simulink model "massignment5"  (Simulink 6.0)
settings: Solver=FixedStepDiscrete  StartTime=0.0  StopTime=10.0  RelTol=1e-3
libraries: massignmentLib x2
settings Model: Creator=awarlock  LastModifiedBy=awarlock  ExtModeAutoUpdateStatusClock=off
settings OptimizationCC: InlineParams=on
settings DebuggingCC: MultiTaskDSMMsg=warning

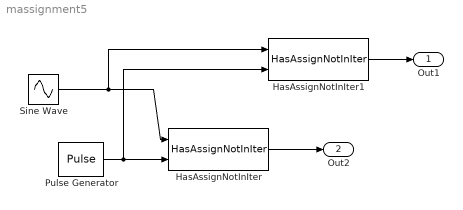
== system massignment5 ==
  HasAssignNotInIter : massignmentLib/HasAssignNotInIter
  HasAssignNotInIter1 : massignmentLib/HasAssignNotInIter
  Pulse Generator : DiscretePulseGenerator  SampleTime=0.1
  Sine Wave : Sin  Amplitude=3:7  SampleTime=0.1
  Out1 : Outport
  Out2 : Outport  Port=2
  wires:
  Sine Wave/1 -> HasAssignNotInIter/1, HasAssignNotInIter1/1
  HasAssignNotInIter1/1 -> Out1/1
  HasAssignNotInIter/1 -> Out2/1
  Pulse Generator/1 -> HasAssignNotInIter/2, HasAssignNotInIter1/2
